simulink model "AudiSim_V3"  (R2023b)
settings: Solver=VariableStepAuto  StartTime=0.0  StopTime=10.0  RelTol=1e-3
values from neighbouring files (symbols this model uses):
  c1 = 86/100    (= 0.86)    [AudiSim_Parameters.m]
  c2 = 33078/1000    (= 33.078)    [AudiSim_Parameters.m]
  c3 = 36/100    (= 0.36)    [AudiSim_Parameters.m]
  Crr = 65/10000    (= 0.0065)    [AudiSim_Parameters.m]
  d = 4953/10000    (= 0.4953)    [AudiSim_Parameters.m]
  g = 981/100    (= 9.81)    [AudiSim_Parameters.m]
  i = 01/10    (= 0.1)    [AudiSim_Parameters.m]
  J = 1    [AudiSim_Parameters.m]
  kd = 8724/1000    (= 8.724)    [AudiSim_Parameters.m]
  m = 2145    [AudiSim_Parameters.m]
  T = 545    [AudiSim_Parameters.m]
  t_goal = 67/10    (= 6.7)    [AudiSim_Parameters.m]
  xd0 = 0    [AudiSim_Parameters.m]
  xd_goal = 277165/10000    (= 27.7165)    [AudiSim_Parameters.m]
settings Model: Creator=BeanieBabyJ  LastModifiedBy=BeanieBabyJ

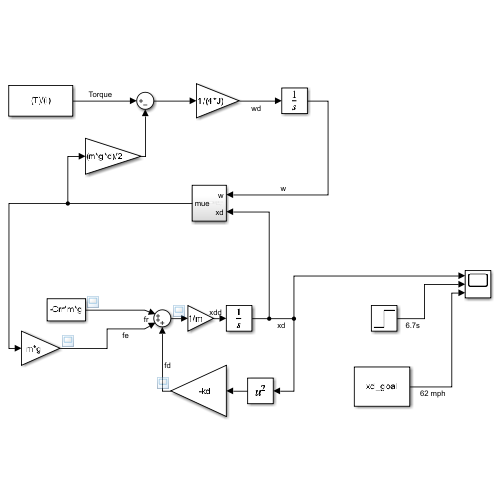
[thumbnail: Simulink's stored preview of the top-level diagram]
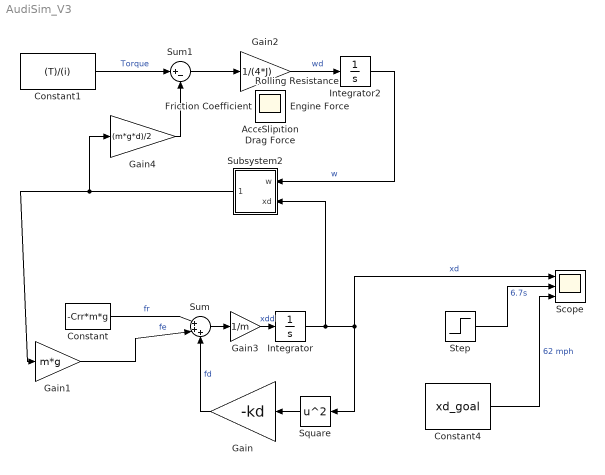
== system AudiSim_V3 ==
  Constant : Constant  Value=-Crr*m*g
  Constant1 : Constant  Value=(T)/(i)
  Constant4 : Constant  Value=xd_goal
  Gain : Gain  Gain=-kd
  Gain1 : Gain  Gain=m*g
  Gain2 : Gain  Gain=1/(4*J)
  Gain3 : Gain  Gain=1/m
  Gain4 : Gain  Gain=(m*g*d)/2
  Integrator : Integrator  InitialCondition=xd0
  Integrator2 : Integrator  InitialCondition=0.1
  Scope : Scope  NumInputPorts=3
  Square : Math  Operator=square
  Step : Step  Time=t_goal  After=xd_goal  SampleTime=0
  Subsystem2 : Subsystem
  Sum : Sum  Inputs=|+++
  Sum1 : Sum  Inputs=|+-
  Acceleration : Scope
  Drag Force : Scope
  Engine Force : Scope
  Friction Coefficient : Scope
  Rolling Resistance : Scope
  Slip : Scope
  wires:
  Constant/1 -> Sum/1  "fr"
  Gain/1 -> Sum/3  "fd"
  Integrator/1 -> Subsystem2/2(xd), Scope/1, Square/1  "xd"
  Square/1 -> Gain/1
  Sum/1 -> Gain3/1
  Gain1/1 -> Sum/2  "fe"
  Constant4/1 -> Scope/3  "62 mph"
  Step/1 -> Scope/2  "6.7s"
  Constant1/1 -> Sum1/1  "Torque"
  Gain3/1 -> Integrator/1  "xdd"
  Subsystem2/1(mue) -> Gain4/1, Gain1/1
  Sum1/1 -> Gain2/1
  Gain2/1 -> Integrator2/1  "wd"
  Integrator2/1 -> Subsystem2/1(w)  "w"
  Gain4/1 -> Sum1/2

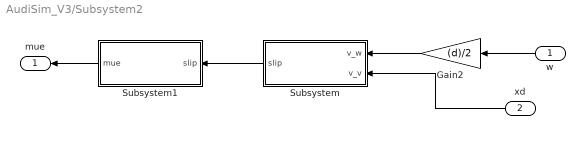
== system AudiSim_V3/Subsystem2 ==
  w : Inport
  xd : Inport  Port=2
  Gain2 : Gain  Gain=(d)/2
  Subsystem : Subsystem
  Subsystem1 : Subsystem
  mue : Outport
  wires:
  Gain2/1 -> Subsystem/1(v_w)
  Subsystem/1(slip) -> Subsystem1/1(slip)
  Subsystem1/1(mue) -> mue/1
  xd/1 -> Subsystem/2(v_v)
  w/1 -> Gain2/1

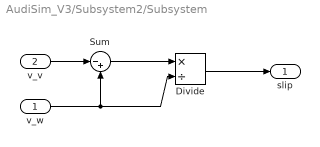
== system AudiSim_V3/Subsystem2/Subsystem ==
  v_w : Inport
  v_v : Inport  Port=2
  Divide : Product  Inputs=*/
  Sum : Sum  Inputs=|-+
  slip : Outport
  wires:
  Sum/1 -> Divide/1
  Divide/1 -> slip/1
  v_v/1 -> Sum/1
  v_w/1 -> Sum/2, Divide/2

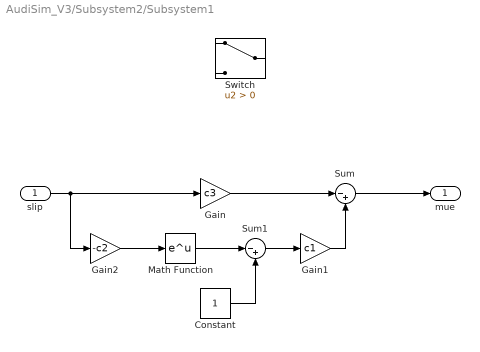
== system AudiSim_V3/Subsystem2/Subsystem1 ==
  slip : Inport
  Constant : Constant
  Gain : Gain  Gain=c3
  Gain1 : Gain  Gain=c1
  Gain2 : Gain  Gain=-c2
  Math Function : Math
  Sum : Sum  Inputs=|-+
  Sum1 : Sum  Inputs=|-+
  Switch : Switch  Criteria=u2 > Threshold  SaturateOnIntegerOverflow=off  InputSameDT=off
  mue : Outport
  wires:
  Sum1/1 -> Gain1/1
  slip/1 -> Gain/1, Gain2/1
  Gain2/1 -> Math Function/1
  Math Function/1 -> Sum1/1
  Constant/1 -> Sum1/2
  Gain1/1 -> Sum/2
  Gain/1 -> Sum/1
  Sum/1 -> mue/1
